simulink model "Stopwatch1"  (Simulink 8.7)
settings: Solver=FixedStepDiscrete  StartTime=0.0  StopTime=100000.0  RelTol=1e-3
settings Model: Creator=scaife  LastModifiedBy=hamza  ExtModeAutoUpdateStatusClock=off
settings DataIOCC: SignalLoggingSaveFormat=ModelDataLogs  SignalLoggingName=sigsOut
settings DebuggingCC: SaveWithParameterizedLinksMsg=none  SignalResolutionControl=TryResolveAllWithWarning  MultiTaskDSMMsg=warning  MultiTaskCondExecSysMsg=none  StrictBusMsg=None
settings HardwareCC: TargetUnknown=on
settings SFSimCC: SimParseCustomCode=off
settings GRTTargetCC: GeneratePreprocessorConditionals=Use local settings  CombineOutputUpdateFcns=off  GRTInterface=on

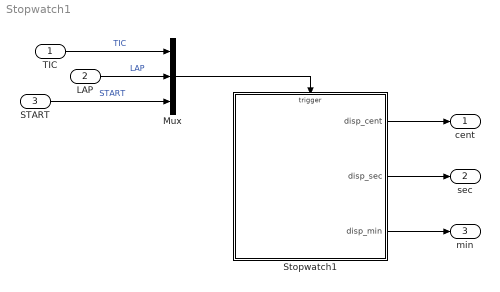
== system Stopwatch1 ==
  TIC : Inport
  LAP : Inport  Port=2
  START : Inport  Port=3
  Mux : Mux  Inputs=3
  Stopwatch1 : Stateflow chart  TreatAsAtomicUnit=on
  cent : Outport
  sec : Outport  Port=2
  min : Outport  Port=3
  wires:
  Stopwatch1/1(disp_cent) -> cent/1
  Stopwatch1/2(disp_sec) -> sec/1
  Stopwatch1/3(disp_min) -> min/1
  TIC/1 -> Mux/1  "TIC"
  LAP/1 -> Mux/2  "LAP"
  Mux/1 -> Stopwatch1/Trigger
  START/1 -> Mux/3  "START"

== stateflow chart Stopwatch1 ==
  state Stopwatch
    state Stop
      state Reset/
        en: runlap=1;
        on LAP:
        cent=0; sec=0; min=0;
        disp_cent=0; disp_sec=0;
        disp_min=0;
      state Lap_stop/
        en: runlap=2;
      (default) -> Reset [order 1] : [runlap==1]
      Lap_stop -> Reset : LAP
      (default) -> Lap_stop [order 2] : [runlap==2]
    state Run
      state Watch [parallel]
        settings: executionOrder=2
        state Running/
          en: runlap=1;
          du:
          disp_cent=cent;
          disp_sec=sec;
          disp_min=min;
        state Lap/
          en: runlap=2;
        (default) -> Running [order 1] : [runlap==1]
        Lap -> Running : LAP
        Running -> Lap : LAP
        (default) -> Lap [order 2] : [runlap==2]
      state Tick [parallel]
        settings: executionOrder=1
        state TicStart
        (default) -> TicStart
        TicStart -> (junction 17) : TIC{cent++;}
        (junction 17) -> (junction 19) [order 2]
        (junction 17) -> (junction 18) [order 1] : [cent==100]{cent=0; sec++;}
        (junction 18) -> (junction 19) [order 2]
        (junction 18) -> (junction 19) [order 1] : [sec==60]{sec=0; min++;}
    (default) -> Stop : {runlap=1;}
    Stop -> Run : START
    Run -> Stop : START
  (default) -> Stopwatch
  data: runlap local int32 =1; cent local int32; sec local int32; min local int32; disp_cent output int32; disp_sec output int32; disp_min output int32
  events: TIC input EITHER_EDGE_EVENT; LAP input EITHER_EDGE_EVENT; START input EITHER_EDGE_EVENT
